simulink library "libturbines"  (R2025b)
settings: Solver=ode45  StartTime=0.0  StopTime=10.0  RelTol=1e-3  EnableMultiTasking=on
undefined symbols (not defined in the file): DiscIntNeverNeededParam, dt, faultOptions, noiseFlag
libraries: simulink x57, $bdroot x3
(part 2 of 5)

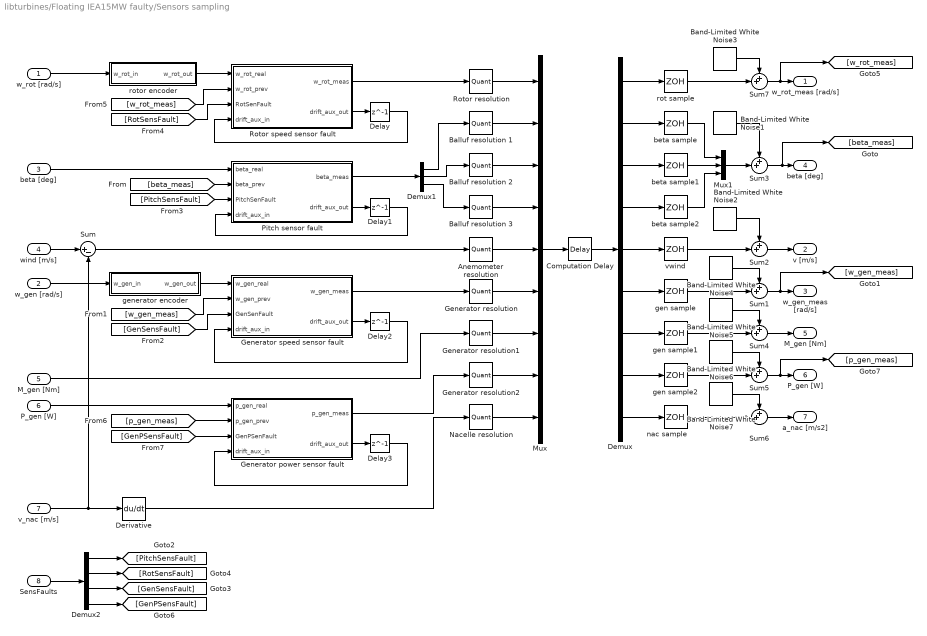
== system libturbines/Floating IEA15MW faulty/Sensors sampling ==
  "w_rot [rad/s] " : Inport
  w_gen [rad/s] : Inport  Port=2
  "beta [deg] " : Inport  Port=3
  wind [m/s] : Inport  Port=4
  "M_gen [Nm] " : Inport  Port=5
  "P_gen [W] " : Inport  Port=6
  "v_nac [m/s] " : Inport  Port=7
  SensFaults : Inport  Port=8
  Anemometer resolution : Quantizer  QuantizationInterval=wt.meas.aneres
  Balluf resolution 1 : Quantizer  QuantizationInterval=wt.meas.pitchres
  Balluf resolution 2 : Quantizer  QuantizationInterval=wt.meas.pitchres
  Balluf resolution 3 : Quantizer  QuantizationInterval=wt.meas.pitchres
  Band-Limited White Noise1 : simulink/Sources/Band-Limited White Noise  Cov=noiseFlag*wt.meas.pitchnoise  Ts=dt  seed=floor(10000*rand(1,3))
  Band-Limited White Noise2 : simulink/Sources/Band-Limited White Noise  Cov=noiseFlag*wt.meas.anenoise  Ts=dt  seed=floor(10000*rand(1))
  Band-Limited White Noise3 : simulink/Sources/Band-Limited White Noise  Cov=noiseFlag*wt.meas.rotSpdnoise  Ts=dt  seed=floor(10000*rand(1))
  Band-Limited White Noise4 : simulink/Sources/Band-Limited White Noise  Cov=noiseFlag*wt.meas.genSpdnoise  Ts=dt  seed=floor(10000*rand(1))
  Band-Limited White Noise5 : simulink/Sources/Band-Limited White Noise  Cov=noiseFlag*wt.meas.genTrqnoise  Ts=dt  seed=floor(10000*rand(1))
  Band-Limited White Noise6 : simulink/Sources/Band-Limited White Noise  Cov=noiseFlag*wt.meas.genPwrnoise  Ts=dt  seed=floor(10000*rand(1))
  Band-Limited White Noise7 : simulink/Sources/Band-Limited White Noise  Cov=noiseFlag*wt.meas.nacAccnoise  Ts=dt  seed=floor(10000*rand(1))
  Computation Delay : TransportDelay  DelayTime=wt.meas.delay  InitialOutput=[wt.rotor.ini wt.pitch.ini wt.pitch.ini wt.pitch.ini 0 wt.gen.ini 0 0 0]
  Delay{,1..3} (4 alike) : Delay  DelayLength=1  InitialCondition=0
  Demux : Demux  Outputs=9
  Demux1 : Demux  Outputs=3
  Demux2 : Demux
  Derivative : Derivative
  Generator power sensor fault : MATLAB Function  TreatAsAtomicUnit=on
  Generator resolution : Quantizer  QuantizationInterval=wt.meas.genres
  Generator resolution1 : Quantizer  QuantizationInterval=wt.meas.genres
  Generator resolution2 : Quantizer  QuantizationInterval=wt.meas.genres
  Generator speed sensor fault : MATLAB Function  TreatAsAtomicUnit=on
  Mux : Mux  Inputs=9
  Mux1 : Mux  Inputs=3
  Nacelle resolution : Quantizer  QuantizationInterval=wt.meas.nacres
  Pitch sensor fault : MATLAB Function  TreatAsAtomicUnit=on
  Rotor resolution : Quantizer  QuantizationInterval=wt.meas.rotres
  Rotor speed sensor fault : MATLAB Function  TreatAsAtomicUnit=on
  Sum : Sum  Inputs=|+-
  Sum{1..7} (7 alike) : Sum  Inputs=++|
  beta sample : ZeroOrderHold  SampleTime=wt.meas.Ts
  beta sample1 : ZeroOrderHold  SampleTime=wt.meas.Ts
  beta sample2 : ZeroOrderHold  SampleTime=wt.meas.Ts
  gen sample : ZeroOrderHold  SampleTime=wt.meas.Ts
  gen sample1 : ZeroOrderHold  SampleTime=wt.meas.Ts
  gen sample2 : ZeroOrderHold  SampleTime=wt.meas.Ts
  generator encoder : Subsystem
  nac sample : ZeroOrderHold  SampleTime=wt.meas.Ts
  rot sample : ZeroOrderHold  SampleTime=wt.meas.Ts
  rotor encoder : Subsystem
  vwind : ZeroOrderHold  SampleTime=wt.meas.Ts
  w_rot_meas [rad/s] : Outport  InitialOutput=0
  v [m/s] : Outport  Port=2  InitialOutput=0
  w_gen_meas [rad/s] : Outport  Port=3  InitialOutput=0
  beta [deg] : Outport  Port=4  InitialOutput=0
  M_gen [Nm] : Outport  Port=5  InitialOutput=0
  P_gen [W] : Outport  Port=6  InitialOutput=0
  a_nac [m/s2] : Outport  Port=7  InitialOutput=0
  wires:
  [p_gen_meas] -> Generator power sensor fault/2(p_gen_prev)
  Generator power sensor fault/1(p_gen_meas) -> Generator resolution2/1
  "P_gen [W] "/1 -> Generator power sensor fault/1(p_gen_real)
  Generator power sensor fault/2(drift_aux_out) -> Delay3/1
  [GenPSensFault] -> Generator power sensor fault/3(GenPSenFault)
  Delay3/1 -> Generator power sensor fault/4(drift_aux_in)
  Demux2/4 -> [GenPSensFault]
  wind [m/s]/1 -> Sum/1
  Sum/1 -> Anemometer resolution/1
  Band-Limited White Noise3/1 -> Sum7/1
  Band-Limited White Noise1/1 -> Sum3/1
  Band-Limited White Noise2/1 -> Sum2/1
  Band-Limited White Noise4/1 -> Sum1/1
  Sum7/1 -> w_rot_meas [rad/s]/1, [w_rot_meas]
  rot sample/1 -> Sum7/2
  Sum3/1 -> beta [deg]/1, [beta_meas]
  Mux1/1 -> Sum3/2
  vwind/1 -> Sum2/2
  Sum2/1 -> v [m/s]/1
  gen sample/1 -> Sum1/2
  Sum1/1 -> w_gen_meas [rad/s]/1, [w_gen_meas]
  Demux/9 -> nac sample/1
  Demux/8 -> gen sample2/1
  Demux/7 -> gen sample1/1
  gen sample2/1 -> Sum5/2
  Sum5/1 -> P_gen [W]/1, [p_gen_meas]
  gen sample1/1 -> Sum4/2
  nac sample/1 -> Sum6/2
  Band-Limited White Noise6/1 -> Sum5/1
  Band-Limited White Noise7/1 -> Sum6/1
  Sum6/1 -> a_nac [m/s2]/1
  Sum4/1 -> M_gen [Nm]/1
  Band-Limited White Noise5/1 -> Sum4/1
  Generator resolution2/1 -> Mux/8
  Nacelle resolution/1 -> Mux/9
  Generator resolution1/1 -> Mux/7
  Derivative/1 -> Nacelle resolution/1
  "v_nac [m/s] "/1 -> Sum/2, Derivative/1
  "M_gen [Nm] "/1 -> Generator resolution1/1
  Delay2/1 -> Generator speed sensor fault/4(drift_aux_in)
  Generator speed sensor fault/2(drift_aux_out) -> Delay2/1
  Delay1/1 -> Pitch sensor fault/4(drift_aux_in)
  Pitch sensor fault/2(drift_aux_out) -> Delay1/1
  Delay/1 -> Rotor speed sensor fault/4(drift_aux_in)
  Rotor speed sensor fault/2(drift_aux_out) -> Delay/1
  Demux2/3 -> [GenSensFault]
  Demux2/2 -> [RotSensFault]
  [w_rot_meas] -> Rotor speed sensor fault/2(w_rot_prev)
  [RotSensFault] -> Rotor speed sensor fault/3(RotSenFault)
  [PitchSensFault] -> Pitch sensor fault/3(PitchSenFault)
  [GenSensFault] -> Generator speed sensor fault/3(GenSenFault)
  Demux2/1 -> [PitchSensFault]
  SensFaults/1 -> Demux2/1
  rotor encoder/1(w_rot_out) -> Rotor speed sensor fault/1(w_rot_real)
  Rotor speed sensor fault/1(w_rot_meas) -> Rotor resolution/1
  "w_rot [rad/s] "/1 -> rotor encoder/1(w_rot_in)
  generator encoder/1(w_gen_out) -> Generator speed sensor fault/1(w_gen_real)
  w_gen [rad/s]/1 -> generator encoder/1(w_gen_in)
  [beta_meas] -> Pitch sensor fault/2(beta_prev)
  [w_gen_meas] -> Generator speed sensor fault/2(w_gen_prev)
  Generator speed sensor fault/1(w_gen_meas) -> Generator resolution/1
  Balluf resolution 3/1 -> Mux/4
  Balluf resolution 2/1 -> Mux/3
  Demux/3 -> beta sample1/1
  Demux/4 -> beta sample2/1
  "beta [deg] "/1 -> Pitch sensor fault/1(beta_real)
  Pitch sensor fault/1(beta_meas) -> Demux1/1
  Balluf resolution 1/1 -> Mux/2
  Demux/2 -> beta sample/1
  beta sample2/1 -> Mux1/3
  Demux/1 -> rot sample/1
  beta sample/1 -> Mux1/1
  Demux1/3 -> Balluf resolution 3/1
  Computation Delay/1 -> Demux/1
  Mux/1 -> Computation Delay/1
  Demux/5 -> vwind/1
  Anemometer resolution/1 -> Mux/5
  Demux/6 -> gen sample/1
  Demux1/2 -> Balluf resolution 2/1
  Generator resolution/1 -> Mux/6
  Rotor resolution/1 -> Mux/1
  Demux1/1 -> Balluf resolution 1/1
  beta sample1/1 -> Mux1/2

== system libturbines/Floating IEA15MW faulty/Tower deflection  ==
  F_t [N] : Inport
  F_t*h : Gain  Gain=wt.tower.height  SaturateOnIntegerOverflow=on  OutDataTypeStr=Inherit: Same as input  ParamDataTypeStr=Inherit: Same as input
  Tower1 : Subsystem  mask(Tower (thrustwise)){mtop=wt.top.mass, mtow=wt.tower.mass, ftowY=wt.tower.eigfreq, dampY=wt.tower.damp}
      mask prompts: mtop "Mass of towertop [kg]"; mtow "Aequivalent tower mass [kg]"; ftowY "Tower eigenfrequency [Hz]"; dampY "Damping coefficient"
      mask help: Thrustwise dynamics of the tower
      mask init: same as libturbines/Floating IEA15MW/Tower /Tower1
      mask Help: The thrustwise tower dynamics are modelled as a linear oscillator
  v_nac [m/s] : Outport
  M_tow [Nm] : Outport  Port=2
  wires:
  Tower1/1(vnac [m/s]) -> v_nac [m/s]/1
  F_t [N]/1 -> Tower1/1(FT [Nm])
  F_t*h/1 -> M_tow [Nm]/1
  Tower1/2(F_tow [N]) -> F_t*h/1

== system libturbines/Floating IEA3.4MW/Aerodynamics ==
  note: tip speed
      | [m/s]
  w_rot [rad/s] : Inport
  beta [deg] : Inport  Port=2
  v_rot [m/s] : Inport  Port=3
  C_P & C_T tables1 : $bdroot/Floating NREL5MW faulty/Aerodynamics/Blade 1/C_P & C_T tables  SystemSampleTime=-1  VariantActivationTime=update diagram  EmptyChoice=off  PassThrough=off  PassThroughVariantControl=(default)  EmptyChoiceVariantControl=(default)  AllowFlexibleInterface=on  Latency=0  AutoFrameSizeCalculation=off
  Math Function : Math  Operator=square  SignedPower=on
  Product : Product  InputSameDT=on  SaturateOnIntegerOverflow=on  OutDataTypeStr=Inherit: Same as first input
  Product1 : Product  Inputs=**/  InputSameDT=on  SaturateOnIntegerOverflow=on  OutDataTypeStr=Inherit: Same as first input
  Product2 : Product  InputSameDT=on  SaturateOnIntegerOverflow=on  OutDataTypeStr=Inherit: Same as first input
  Product3 : Product  Inputs=/*  InputSameDT=on  SaturateOnIntegerOverflow=on  OutDataTypeStr=Inherit: Same as first input
  rho/2*A : Gain  Gain=env.rho*.5* pi * wt.rotor.radius^2  SaturateOnIntegerOverflow=on  OutDataTypeStr=Inherit: Same as input  ParamDataTypeStr=Inherit: Same as input
  rotor radius : Gain  Gain=wt.rotor.radius  SaturateOnIntegerOverflow=on  OutDataTypeStr=Inherit: Same as input  ParamDataTypeStr=Inherit: Same as input
  M_rot [Nm] : Outport
  F_t [N] : Outport  Port=2
  C_T : Outport  Port=3
  wires:
  rho/2*A/1 -> Product/1, Product2/2
  C_P & C_T tables1/1 -> Product/2, C_T/1
  Product3/1 -> C_P & C_T tables1/2
  w_rot [rad/s]/1 -> Product1/3, rotor radius/1
  v_rot [m/s]/1 -> Product2/1, Product3/1, Math Function/1
  Math Function/1 -> rho/2*A/1
  rotor radius/1 -> Product3/2
  C_P & C_T tables1/2 -> Product1/1
  beta [deg]/1 -> C_P & C_T tables1/1
  Product/1 -> F_t [N]/1
  Product1/1 -> M_rot [Nm]/1
  Product2/1 -> Product1/2

== system libturbines/Floating IEA3.4MW/Controller ==
  P_dem [W] : Inport
  w_gen_meas [m/s] : Inport  Port=2
  beta_meas [deg] : Inport  Port=3
  Generator efficiency compensation : Gain  Gain=1/wt.ctrl.gen.effeciency
  Limit power to rated : Saturate  UpperLimit=wt.ctrl.p_rated  LowerLimit=0
  Measurement filter (low pass) : DiscreteStateSpace  A=wt.ctrl.alpha  B=1-wt.ctrl.alpha  C=wt.ctrl.alpha  D=1-wt.ctrl.alpha  InitialCondition=wt.ctrl.gen.ini  SampleTime=wt.ctrl.Ts
  Pitch controller : Subsystem  TreatAsAtomicUnit=on
  Rate Limiter : RateLimiter  RisingSlewLimit=wt.ctrl.torq.ratelim  FallingSlewLimit=-wt.ctrl.torq.ratelim  SampleTimeMode=inherited  InitialCondition=wt.ctrl.torq.ini
  Rated speed : Constant  Value=wt.ctrl.gen.rated
  Region check : Subsystem
  Sample output : ZeroOrderHold  SampleTime=wt.ctrl.Ts
  Sample power demand : ZeroOrderHold  SampleTime=wt.ctrl.Ts
  Saturation : Saturate  UpperLimit=wt.ctrl.torq.lim  LowerLimit=0
  Sum : Sum  Inputs=+-|
  Torque - speed lookup table : Lookup  InputValues=wt.ctrl.torq.wg  Table=wt.ctrl.torq.M  LookUpMeth=Interpolation-Use End Values  SaturateOnIntegerOverflow=off
  Zero-Order Hold : ZeroOrderHold  SampleTime=wt.ctrl.Ts
  beta_ref [deg] : Outport
  M_g_ref [W] : Outport  Port=2
  wires:
  Region check/2(Enable pitch controller) -> Pitch controller/Enable
  Sum/1 -> Pitch controller/1(w_gen_diff)
  Rated speed/1 -> Sum/1
  Sample power demand/1 -> Generator efficiency compensation/1
  Rate Limiter/1 -> Sample output/1
  Generator efficiency compensation/1 -> Limit power to rated/1
  Sample output/1 -> M_g_ref [W]/1
  Zero-Order Hold/1 -> beta_ref [deg]/1
  Limit power to rated/1 -> Region check/3(p_dem), Pitch controller/2(P_dem)
  Region check/1(Torque_ref) -> Saturation/1
  P_dem [W]/1 -> Sample power demand/1
  Torque - speed lookup table/1 -> Region check/1(Torque_dem)  "Desired Torque"
  Saturation/1 -> Rate Limiter/1
  Measurement filter (low pass)/1 -> Sum/2, Region check/2(w_gen), Torque - speed lookup table/1  "Filtered generator speed"
  w_gen_meas [m/s]/1 -> Measurement filter (low pass)/1
  Pitch controller/1(beta_ref [deg]) -> Zero-Order Hold/1, Region check/4(pitch command)
  beta_meas [deg]/1 -> Pitch controller/3(beta_meas [deg])

== system libturbines/Floating IEA3.4MW/Drive Train ==
  M_rot [Nm] : Inport
  M_gen [Nm] : Inport  Port=2
  Demux : Demux  Outputs=3
  Drive train dynamics : StateSpace  A=wt.dt.ssA  B=wt.dt.ssB  C=wt.dt.ssC  D=wt.dt.ssD  InitialCondition=[wt.rotor.ini;wt.gen.ini;0]
  Mux : Mux  Inputs=2
  w_rot [rad/s] : Outport
  w_gen [rad/s] : Outport  Port=2
  M_shaft [Nm] : Outport  Port=3
  wires:
  Mux/1 -> Drive train dynamics/1
  M_rot [Nm]/1 -> Mux/1
  M_gen [Nm]/1 -> Mux/2
  Drive train dynamics/1 -> Demux/1
  Demux/1 -> w_rot [rad/s]/1
  Demux/2 -> w_gen [rad/s]/1
  Demux/3 -> M_shaft [Nm]/1

== system libturbines/Floating IEA3.4MW/Generator simple ==
  w_gen [rad/s] : Inport
  M_g_ref [W] : Inport  Port=2
  Constant : Constant  Value=wt.gen.timeconstant
  Divide1 : Product  Inputs=*/
  Generator efficiency : Gain  Gain=wt.gen.effeciency
  Multiply : Product  Inputs=**
  Sum : Sum  Inputs=|+-
  Torque Integrator : Integrator  InitialCondition=wt.gen.torq.ini
  M_gen [Nm] : Outport
  P_out [W] : Outport  Port=2
  wires:
  Constant/1 -> Divide1/2
  Divide1/1 -> Torque Integrator/1
  Generator efficiency/1 -> P_out [W]/1
  Multiply/1 -> Generator efficiency/1
  M_g_ref [W]/1 -> Sum/1
  w_gen [rad/s]/1 -> Multiply/2
  Torque Integrator/1 -> M_gen [Nm]/1, Sum/2, Multiply/1
  Sum/1 -> Divide1/1

== system libturbines/Floating IEA3.4MW/Hydrodynamics ==
  F_t [N] : Inport
  F_ex : Inport  Port=2
  Gain : Gain  Gain=plat.nF2pT  Multiplication=Matrix(K*u)
  Gain2 : Gain  Gain=plat.pM2nM_surge  Multiplication=Matrix(K*u)
  Gain3 : Gain  Gain=plat.pM2nM_pitch  Multiplication=Matrix(K*u)
  Platform hydrodynamics SS system : StateSpace  A=plat.HydSys.a  B=plat.HydSys.b  C=plat.HydSys.c  D=plat.HydSys.d  InitialCondition=0
  Sum : Sum  Inputs=++|
  Sum2 : Sum  Inputs=+|+
  v_nac_hyd [m/s] : Outport
  wires:
  F_ex/1 -> Sum/2
  Sum/1 -> Platform hydrodynamics SS system/1
  Sum2/1 -> v_nac_hyd [m/s]/1
  Platform hydrodynamics SS system/1 -> Gain3/1, Gain2/1
  Gain2/1 -> Sum2/1
  Gain3/1 -> Sum2/2
  Gain/1 -> Sum/1
  F_t [N]/1 -> Gain/1

== system libturbines/Floating IEA3.4MW/Pitch Actuator ==
  beta_ref [deg] : Inport
  Pitch system : StateSpace  A=wt.pitch.ssA  B=wt.pitch.ssB  C=wt.pitch.ssC  D=wt.pitch.ssD  InitialCondition=0
  beta [deg] : Outport
  wires:
  beta_ref [deg]/1 -> Pitch system/1
  Pitch system/1 -> beta [deg]/1

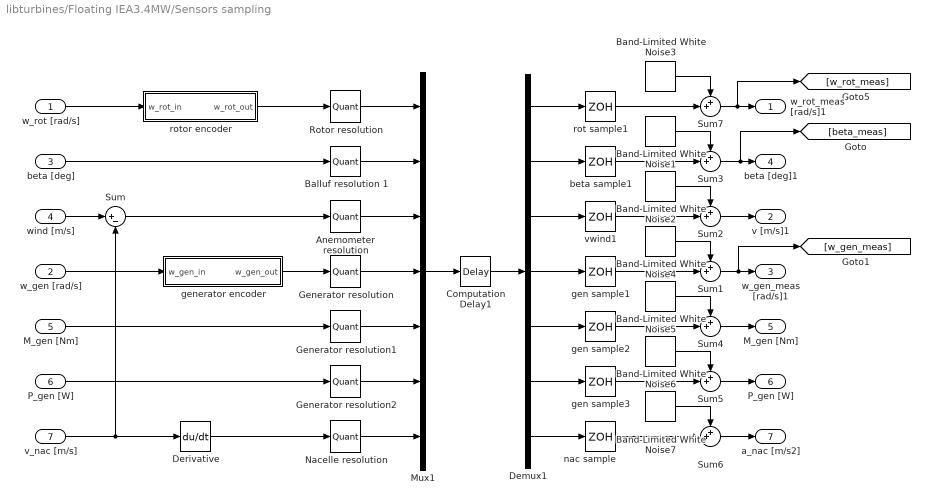
== system libturbines/Floating IEA3.4MW/Sensors sampling ==
  "w_rot [rad/s] " : Inport
  w_gen [rad/s] : Inport  Port=2
  "beta [deg] " : Inport  Port=3
  wind [m/s] : Inport  Port=4
  "M_gen [Nm] " : Inport  Port=5
  "P_gen [W] " : Inport  Port=6
  "v_nac [m/s] " : Inport  Port=7
  Anemometer resolution : Quantizer  QuantizationInterval=wt.meas.aneres
  Balluf resolution 1 : Quantizer  QuantizationInterval=wt.meas.pitchres
  Band-Limited White Noise1 : simulink/Sources/Band-Limited White Noise  Cov=noiseFlag*wt.meas.pitchnoise  Ts=dt  seed=floor(10000*rand(1))
  Band-Limited White Noise2 : simulink/Sources/Band-Limited White Noise  Cov=noiseFlag*wt.meas.anenoise  Ts=dt  seed=floor(10000*rand(1))
  Band-Limited White Noise3 : simulink/Sources/Band-Limited White Noise  Cov=noiseFlag*wt.meas.rotSpdnoise  Ts=dt  seed=floor(10000*rand(1))
  Band-Limited White Noise4 : simulink/Sources/Band-Limited White Noise  Cov=noiseFlag*wt.meas.genSpdnoise  Ts=dt  seed=floor(10000*rand(1))
  Band-Limited White Noise5 : simulink/Sources/Band-Limited White Noise  Cov=noiseFlag*wt.meas.genTrqnoise  Ts=dt  seed=floor(10000*rand(1))
  Band-Limited White Noise6 : simulink/Sources/Band-Limited White Noise  Cov=noiseFlag*wt.meas.genPwrnoise  Ts=dt  seed=floor(10000*rand(1))
  Band-Limited White Noise7 : simulink/Sources/Band-Limited White Noise  Cov=noiseFlag*wt.meas.nacAccnoise  Ts=dt  seed=floor(10000*rand(1))
  Computation Delay1 : TransportDelay  DelayTime=wt.meas.delay  InitialOutput=[wt.rotor.ini wt.pitch.ini 0 wt.gen.ini 0 0 0]
  Demux1 : Demux  Outputs=7
  Derivative : Derivative
  Generator resolution : Quantizer  QuantizationInterval=wt.meas.genres
  Generator resolution1 : Quantizer  QuantizationInterval=wt.meas.genres
  Generator resolution2 : Quantizer  QuantizationInterval=wt.meas.genres
  Mux1 : Mux  Inputs=7
  Nacelle resolution : Quantizer  QuantizationInterval=wt.meas.nacres
  Rotor resolution : Quantizer  QuantizationInterval=wt.meas.rotres
  Sum : Sum  Inputs=|+-
  Sum{1..7} (7 alike) : Sum  Inputs=++|
  beta sample1 : ZeroOrderHold  SampleTime=wt.meas.Ts
  gen sample1 : ZeroOrderHold  SampleTime=wt.meas.Ts
  gen sample2 : ZeroOrderHold  SampleTime=wt.meas.Ts
  gen sample3 : ZeroOrderHold  SampleTime=wt.meas.Ts
  generator encoder : Subsystem
  nac sample : ZeroOrderHold  SampleTime=wt.meas.Ts
  rot sample1 : ZeroOrderHold  SampleTime=wt.meas.Ts
  rotor encoder : Subsystem
  vwind1 : ZeroOrderHold  SampleTime=wt.meas.Ts
  w_rot_meas [rad/s]1 : Outport  InitialOutput=0
  v [m/s]1 : Outport  Port=2  InitialOutput=0
  w_gen_meas [rad/s]1 : Outport  Port=3  InitialOutput=0
  beta [deg]1 : Outport  Port=4  InitialOutput=0
  M_gen [Nm] : Outport  Port=5  InitialOutput=0
  P_gen [W] : Outport  Port=6  InitialOutput=0
  a_nac [m/s2] : Outport  Port=7  InitialOutput=0
  wires:
  Sum/1 -> Anemometer resolution/1
  wind [m/s]/1 -> Sum/1
  "M_gen [Nm] "/1 -> Generator resolution1/1
  "P_gen [W] "/1 -> Generator resolution2/1
  Derivative/1 -> Nacelle resolution/1
  Nacelle resolution/1 -> Mux1/7
  Generator resolution2/1 -> Mux1/6
  Generator resolution1/1 -> Mux1/5
  Demux1/3 -> vwind1/1
  Demux1/4 -> gen sample1/1
  Demux1/5 -> gen sample2/1
  Demux1/6 -> gen sample3/1
  Demux1/7 -> nac sample/1
  "v_nac [m/s] "/1 -> Derivative/1, Sum/2
  Generator resolution/1 -> Mux1/4
  Anemometer resolution/1 -> Mux1/3
  Balluf resolution 1/1 -> Mux1/2
  Band-Limited White Noise2/1 -> Sum2/1
  gen sample2/1 -> Sum4/2
  Sum1/1 -> w_gen_meas [rad/s]1/1, [w_gen_meas]
  Sum5/1 -> P_gen [W]/1
  gen sample3/1 -> Sum5/2
  Band-Limited White Noise1/1 -> Sum3/1
  nac sample/1 -> Sum6/2
  Sum4/1 -> M_gen [Nm]/1
  Sum6/1 -> a_nac [m/s2]/1
  vwind1/1 -> Sum2/2
  Sum7/1 -> w_rot_meas [rad/s]1/1, [w_rot_meas]
  Band-Limited White Noise4/1 -> Sum1/1
  Band-Limited White Noise5/1 -> Sum4/1
  gen sample1/1 -> Sum1/2
  Band-Limited White Noise3/1 -> Sum7/1
  rot sample1/1 -> Sum7/2
  Mux1/1 -> Computation Delay1/1
  Sum3/1 -> beta [deg]1/1, [beta_meas]
  Sum2/1 -> v [m/s]1/1
  Band-Limited White Noise6/1 -> Sum5/1
  Band-Limited White Noise7/1 -> Sum6/1
  Demux1/2 -> beta sample1/1
  Demux1/1 -> rot sample1/1
  beta sample1/1 -> Sum3/2
  Computation Delay1/1 -> Demux1/1
  "beta [deg] "/1 -> Balluf resolution 1/1
  Rotor resolution/1 -> Mux1/1
  generator encoder/1(w_gen_out) -> Generator resolution/1
  w_gen [rad/s]/1 -> generator encoder/1(w_gen_in)
  "w_rot [rad/s] "/1 -> rotor encoder/1(w_rot_in)
  rotor encoder/1(w_rot_out) -> Rotor resolution/1

== system libturbines/Floating IEA3.4MW/Tower  ==
  F_t [N] : Inport
  F_t*h : Gain  Gain=wt.tower.height  SaturateOnIntegerOverflow=on  OutDataTypeStr=Inherit: Same as input  ParamDataTypeStr=Inherit: Same as input
  Tower1 : Subsystem  mask(Tower (thrustwise)){mtop=wt.top.mass, mtow=wt.tower.mass, ftowY=wt.tower.eigfreq, dampY=wt.tower.damp}
      mask prompts: mtop "Mass of towertop [kg]"; mtow "Aequivalent tower mass [kg]"; ftowY "Tower eigenfrequency [Hz]"; dampY "Damping coefficient"
      mask help: Thrustwise dynamics of the tower
      mask init: same as libturbines/Floating IEA15MW/Tower /Tower1
      mask Help: The thrustwise tower dynamics are modelled as a linear oscillator
  M_tow [Nm] : Outport
  v_nac [m/s] : Outport  Port=2
  wires:
  Tower1/2(F_tow [N]) -> F_t*h/1
  F_t*h/1 -> M_tow [Nm]/1
  F_t [N]/1 -> Tower1/1(FT [Nm])
  Tower1/1(vnac [m/s]) -> v_nac [m/s]/1

== system libturbines/Floating IEA3.4MW faulty/Aerodynamics ==
  w_rot [rad/s] : Inport
  beta [deg] : Inport  Port=2
  v_rot [m/s] : Inport  Port=3
  Blade 1 : Subsystem
  Blade 2 : Subsystem  AncestorBlock=libturbines/Floating faulty NREL5MW1/Aerodynamics/Blade 1
  Blade 3 : Subsystem  AncestorBlock=libturbines/Floating faulty NREL5MW1/Aerodynamics/Blade 1
  Demux : Demux  Outputs=3
  Sum : Sum  Inputs=+++
  Sum1 : Sum  Inputs=+++
  Sum2 : Sum  Inputs=+++
  M_rot [Nm] : Outport
  F_t [N] : Outport  Port=2
  C_T : Outport  Port=3
  wires:
  Demux/2 -> Blade 2/2(beta [deg])
  Demux/3 -> Blade 3/2(beta [deg])
  Demux/1 -> Blade 1/2(beta [deg])
  beta [deg]/1 -> Demux/1
  Blade 2/2(C_T) -> Sum1/2
  Blade 2/1(F_t [N]) -> Sum/2
  Blade 1/2(C_T) -> Sum1/1
  Blade 1/1(F_t [N]) -> Sum/1
  Blade 1/3(M_rot [Nm]) -> Sum2/1
  Blade 3/2(C_T) -> Sum1/3
  Blade 3/1(F_t [N]) -> Sum/3
  Blade 3/3(M_rot [Nm]) -> Sum2/3
  Blade 2/3(M_rot [Nm]) -> Sum2/2
  Sum1/1 -> C_T/1
  Sum2/1 -> M_rot [Nm]/1
  Sum/1 -> F_t [N]/1
  w_rot [rad/s]/1 -> Blade 1/3(w_rot [rad/s]), Blade 2/3(w_rot [rad/s]), Blade 3/3(w_rot [rad/s])
  v_rot [m/s]/1 -> Blade 1/1(v_rot [m/s]), Blade 2/1(v_rot [m/s]), Blade 3/1(v_rot [m/s])

== system libturbines/Floating IEA3.4MW faulty/Controller ==
  P_dem [W] : Inport
  w_gen_meas [m/s] : Inport  Port=2
  beta_meas [deg] : Inport  Port=3
  Gain : Gain  Gain=[1 0 0]  Multiplication=Matrix(K*u) (u vector)
  Generator efficiency compensation : Gain  Gain=1/wt.ctrl.gen.effeciency
  Limit power to rated : Saturate  UpperLimit=wt.ctrl.p_rated  LowerLimit=0
  Measurement filter (low pass) : DiscreteStateSpace  A=wt.ctrl.alpha  B=1-wt.ctrl.alpha  C=wt.ctrl.alpha  D=1-wt.ctrl.alpha  InitialCondition=wt.ctrl.gen.ini  SampleTime=wt.ctrl.Ts
  Pitch controller : Subsystem  TreatAsAtomicUnit=on
  Rate Limiter : RateLimiter  RisingSlewLimit=wt.ctrl.torq.ratelim  FallingSlewLimit=-wt.ctrl.torq.ratelim  SampleTimeMode=inherited  InitialCondition=wt.ctrl.torq.ini
  Rated speed : Constant  Value=wt.ctrl.gen.rated
  Region check : Subsystem
  Sample output : ZeroOrderHold  SampleTime=wt.ctrl.Ts
  Sample power demand : ZeroOrderHold  SampleTime=wt.ctrl.Ts
  Saturation : Saturate  UpperLimit=wt.ctrl.torq.lim  LowerLimit=0
  Sum : Sum  Inputs=+-|
  Torque - speed lookup table : Lookup  InputValues=wt.ctrl.torq.wg  Table=wt.ctrl.torq.M  LookUpMeth=Interpolation-Use End Values  SaturateOnIntegerOverflow=off
  Zero-Order Hold : ZeroOrderHold  SampleTime=wt.ctrl.Ts
  beta_ref [deg] : Outport
  T_g_ref [W] : Outport  Port=2
  wires:
  beta_meas [deg]/1 -> Pitch controller/3(beta_meas [deg])
  Gain/1 -> Region check/4(pitch command)
  w_gen_meas [m/s]/1 -> Measurement filter (low pass)/1
  Measurement filter (low pass)/1 -> Torque - speed lookup table/1, Region check/2(w_gen), Sum/2  "Filtered generator speed"
  Saturation/1 -> Rate Limiter/1
  Pitch controller/1(beta_ref [deg]) -> Zero-Order Hold/1, Gain/1
  Torque - speed lookup table/1 -> Region check/1(Torque_dem)  "Desired Torque"
  P_dem [W]/1 -> Sample power demand/1
  Region check/1(Torque_ref) -> Saturation/1
  Limit power to rated/1 -> Pitch controller/2(P_dem), Region check/3(p_dem)
  Zero-Order Hold/1 -> beta_ref [deg]/1
  Sample output/1 -> T_g_ref [W]/1
  Generator efficiency compensation/1 -> Limit power to rated/1
  Rate Limiter/1 -> Sample output/1
  Sample power demand/1 -> Generator efficiency compensation/1
  Rated speed/1 -> Sum/1
  Sum/1 -> Pitch controller/1(w_gen_diff)
  Region check/2(Enable pitch controller) -> Pitch controller/Enable

== system libturbines/Floating IEA3.4MW faulty/Drive Train ==
  M_rot [Nm] : Inport
  M_gen [Nm] : Inport  Port=2
  Demux : Demux  Outputs=3
  Drive train dynamics : StateSpace  A=wt.dt.ssA  B=wt.dt.ssB  C=wt.dt.ssC  D=wt.dt.ssD  InitialCondition=[wt.rotor.ini;wt.gen.ini;0]
  Mux : Mux  Inputs=2
  w_rot [rad/s] : Outport
  w_gen [rad/s] : Outport  Port=2
  M_shaft [Nm] : Outport  Port=3
  wires:
  Demux/3 -> M_shaft [Nm]/1
  Demux/2 -> w_gen [rad/s]/1
  Demux/1 -> w_rot [rad/s]/1
  Drive train dynamics/1 -> Demux/1
  M_gen [Nm]/1 -> Mux/2
  M_rot [Nm]/1 -> Mux/1
  Mux/1 -> Drive train dynamics/1

== system libturbines/Floating IEA3.4MW faulty/Generator simple ==
  w_gen [rad/s] : Inport
  T_g_ref [W] : Inport  Port=2
  GenActFault : Inport  Port=3
  Constant : Constant  Value=wt.gen.timeconstant
  Delay : Delay  DelayLength=1  InitialCondition=0
  Delay1 : Delay  DelayLength=1  InitialCondition=0
  Demux : Demux  Outputs=2
  Divide1 : Product  Inputs=*/
  Generator efficiency : Gain  Gain=wt.gen.effeciency
  Generator fault : MATLAB Function  TreatAsAtomicUnit=on
  Generator fault type 3 : MATLAB Function  TreatAsAtomicUnit=on
  Multiply : Product  Inputs=**
  Product : Product
  Sum : Sum  Inputs=|+-
  Torque Integrator : Integrator  InitialCondition=wt.gen.torq.ini
  M_gen [Nm] : Outport
  P_out [W] : Outport  Port=2
  wires:
  Delay1/1 -> Generator fault/4(drift_aux_in)
  Generator fault/2(drift_aux_out) -> Delay1/1
  Delay/1 -> Generator fault/3(torque_prev)
  Sum/1 -> Divide1/1
  Product/1 -> Divide1/2
  Demux/2 -> Product/1
  Constant/1 -> Product/2
  Generator fault/1(torque_real) -> M_gen [Nm]/1, Delay/1, Multiply/1
  Demux/1 -> Generator fault/1(GenActFault)
  Generator fault type 3/1(out) -> Demux/1
  GenActFault/1 -> Generator fault type 3/1(GenActFault)
  w_gen [rad/s]/1 -> Multiply/2
  Torque Integrator/1 -> Sum/2, Generator fault/2(torque)
  T_g_ref [W]/1 -> Sum/1
  Multiply/1 -> Generator efficiency/1
  Generator efficiency/1 -> P_out [W]/1
  Divide1/1 -> Torque Integrator/1

== system libturbines/Floating IEA3.4MW faulty/Hydrodynamics ==
  F_t [N] : Inport
  F_ex : Inport  Port=2
  Gain : Gain  Gain=plat.nF2pT  Multiplication=Matrix(K*u)
  Gain2 : Gain  Gain=plat.pM2nM_surge  Multiplication=Matrix(K*u)
  Gain3 : Gain  Gain=plat.pM2nM_pitch  Multiplication=Matrix(K*u)
  Platform hydrodynamics SS system : StateSpace  A=plat.HydSys.a  B=plat.HydSys.b  C=plat.HydSys.c  D=plat.HydSys.d  InitialCondition=0
  Sum : Sum  Inputs=++|
  Sum2 : Sum  Inputs=+|+
  v_nac_hyd [m/s] : Outport
  wires:
  F_t [N]/1 -> Gain/1
  Gain/1 -> Sum/1
  Gain3/1 -> Sum2/2
  Gain2/1 -> Sum2/1
  Platform hydrodynamics SS system/1 -> Gain2/1, Gain3/1
  Sum2/1 -> v_nac_hyd [m/s]/1
  Sum/1 -> Platform hydrodynamics SS system/1
  F_ex/1 -> Sum/2

== system libturbines/Floating IEA3.4MW faulty/Pitch Actuator ==
  beta_ref [deg] : Inport
  PitchActFault : Inport  Port=2
  Delay1 : Delay  DelayLength=1  InitialCondition=0
  Delay2 : Delay  DelayLength=1  InitialCondition=0
  Pitch actuator fault : MATLAB Function  TreatAsAtomicUnit=on
  Pitch subsystems : Subsystem
  beta [deg] : Outport
  wires:
  Delay1/1 -> Pitch actuator fault/2(beta_prev)
  Delay2/1 -> Pitch actuator fault/4(drift_aux_in)
  Pitch actuator fault/2(drift_aux_out) -> Delay2/1
  Pitch subsystems/1(beta [deg]) -> Pitch actuator fault/1(beta)
  Pitch actuator fault/1(beta_real) -> beta [deg]/1, Delay1/1
  beta_ref [deg]/1 -> Pitch subsystems/1(beta_ref [deg])
  PitchActFault/1 -> Pitch actuator fault/3(PitchActFault), Pitch subsystems/2(Fault type 5)

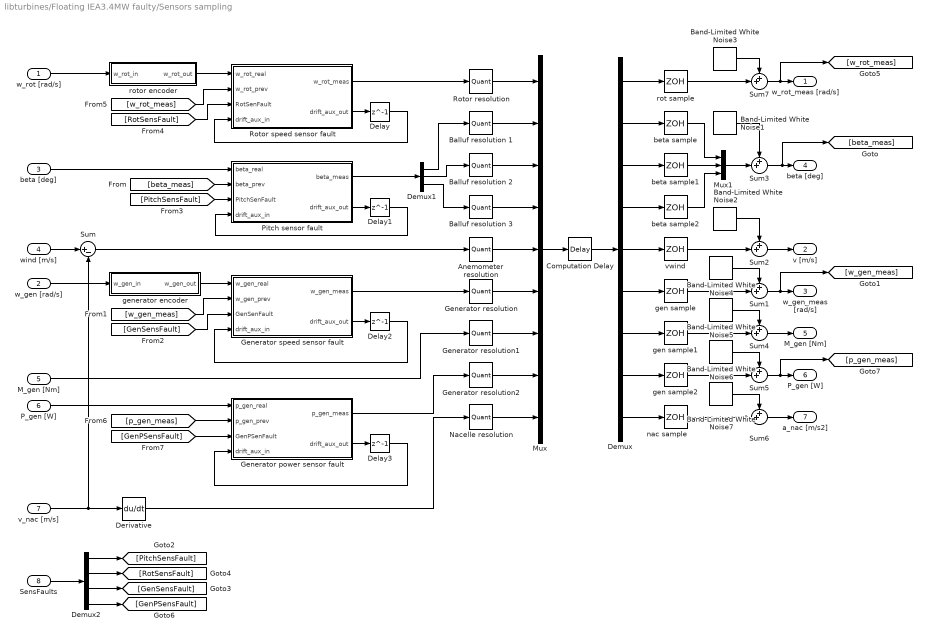
== system libturbines/Floating IEA3.4MW faulty/Sensors sampling ==
  "w_rot [rad/s] " : Inport
  w_gen [rad/s] : Inport  Port=2
  "beta [deg] " : Inport  Port=3
  wind [m/s] : Inport  Port=4
  "M_gen [Nm] " : Inport  Port=5
  "P_gen [W] " : Inport  Port=6
  "v_nac [m/s] " : Inport  Port=7
  SensFaults : Inport  Port=8
  Anemometer resolution : Quantizer  QuantizationInterval=wt.meas.aneres
  Balluf resolution 1 : Quantizer  QuantizationInterval=wt.meas.pitchres
  Balluf resolution 2 : Quantizer  QuantizationInterval=wt.meas.pitchres
  Balluf resolution 3 : Quantizer  QuantizationInterval=wt.meas.pitchres
  Band-Limited White Noise1 : simulink/Sources/Band-Limited White Noise  Cov=noiseFlag*wt.meas.pitchnoise  Ts=dt  seed=floor(10000*rand(1,3))
  Band-Limited White Noise2 : simulink/Sources/Band-Limited White Noise  Cov=noiseFlag*wt.meas.anenoise  Ts=dt  seed=floor(10000*rand(1))
  Band-Limited White Noise3 : simulink/Sources/Band-Limited White Noise  Cov=noiseFlag*wt.meas.rotSpdnoise  Ts=dt  seed=floor(10000*rand(1))
  Band-Limited White Noise4 : simulink/Sources/Band-Limited White Noise  Cov=noiseFlag*wt.meas.genSpdnoise  Ts=dt  seed=floor(10000*rand(1))
  Band-Limited White Noise5 : simulink/Sources/Band-Limited White Noise  Cov=noiseFlag*wt.meas.genTrqnoise  Ts=dt  seed=floor(10000*rand(1))
  Band-Limited White Noise6 : simulink/Sources/Band-Limited White Noise  Cov=noiseFlag*wt.meas.genPwrnoise  Ts=dt  seed=floor(10000*rand(1))
  Band-Limited White Noise7 : simulink/Sources/Band-Limited White Noise  Cov=noiseFlag*wt.meas.nacAccnoise  Ts=dt  seed=floor(10000*rand(1))
  Computation Delay : TransportDelay  DelayTime=wt.meas.delay  InitialOutput=[wt.rotor.ini wt.pitch.ini wt.pitch.ini wt.pitch.ini 0 wt.gen.ini 0 0 0]
  Delay{,1..3} (4 alike) : Delay  DelayLength=1  InitialCondition=0
  Demux : Demux  Outputs=9
  Demux1 : Demux  Outputs=3
  Demux2 : Demux
  Derivative : Derivative
  Generator power sensor fault : MATLAB Function  TreatAsAtomicUnit=on
  Generator resolution : Quantizer  QuantizationInterval=wt.meas.genres
  Generator resolution1 : Quantizer  QuantizationInterval=wt.meas.genres
  Generator resolution2 : Quantizer  QuantizationInterval=wt.meas.genres
  Generator speed sensor fault : MATLAB Function  TreatAsAtomicUnit=on
  Mux : Mux  Inputs=9
  Mux1 : Mux  Inputs=3
  Nacelle resolution : Quantizer  QuantizationInterval=wt.meas.nacres
  Pitch sensor fault : MATLAB Function  TreatAsAtomicUnit=on
  Rotor resolution : Quantizer  QuantizationInterval=wt.meas.rotres
  Rotor speed sensor fault : MATLAB Function  TreatAsAtomicUnit=on
  Sum : Sum  Inputs=|+-
  Sum{1..7} (7 alike) : Sum  Inputs=++|
  beta sample : ZeroOrderHold  SampleTime=wt.meas.Ts
  beta sample1 : ZeroOrderHold  SampleTime=wt.meas.Ts
  beta sample2 : ZeroOrderHold  SampleTime=wt.meas.Ts
  gen sample : ZeroOrderHold  SampleTime=wt.meas.Ts
  gen sample1 : ZeroOrderHold  SampleTime=wt.meas.Ts
  gen sample2 : ZeroOrderHold  SampleTime=wt.meas.Ts
  generator encoder : Subsystem
  nac sample : ZeroOrderHold  SampleTime=wt.meas.Ts
  rot sample : ZeroOrderHold  SampleTime=wt.meas.Ts
  rotor encoder : Subsystem
  vwind : ZeroOrderHold  SampleTime=wt.meas.Ts
  w_rot_meas [rad/s] : Outport  InitialOutput=0
  v [m/s] : Outport  Port=2  InitialOutput=0
  w_gen_meas [rad/s] : Outport  Port=3  InitialOutput=0
  beta [deg] : Outport  Port=4  InitialOutput=0
  M_gen [Nm] : Outport  Port=5  InitialOutput=0
  P_gen [W] : Outport  Port=6  InitialOutput=0
  a_nac [m/s2] : Outport  Port=7  InitialOutput=0
  wires:
  [p_gen_meas] -> Generator power sensor fault/2(p_gen_prev)
  Generator power sensor fault/1(p_gen_meas) -> Generator resolution2/1
  "P_gen [W] "/1 -> Generator power sensor fault/1(p_gen_real)
  Generator power sensor fault/2(drift_aux_out) -> Delay3/1
  [GenPSensFault] -> Generator power sensor fault/3(GenPSenFault)
  Delay3/1 -> Generator power sensor fault/4(drift_aux_in)
  Demux2/4 -> [GenPSensFault]
  wind [m/s]/1 -> Sum/1
  Sum/1 -> Anemometer resolution/1
  Band-Limited White Noise3/1 -> Sum7/1
  Band-Limited White Noise1/1 -> Sum3/1
  Band-Limited White Noise2/1 -> Sum2/1
  Band-Limited White Noise4/1 -> Sum1/1
  Sum7/1 -> w_rot_meas [rad/s]/1, [w_rot_meas]
  rot sample/1 -> Sum7/2
  Sum3/1 -> beta [deg]/1, [beta_meas]
  Mux1/1 -> Sum3/2
  vwind/1 -> Sum2/2
  Sum2/1 -> v [m/s]/1
  gen sample/1 -> Sum1/2
  Sum1/1 -> w_gen_meas [rad/s]/1, [w_gen_meas]
  Demux/9 -> nac sample/1
  Demux/8 -> gen sample2/1
  Demux/7 -> gen sample1/1
  gen sample2/1 -> Sum5/2
  Sum5/1 -> P_gen [W]/1, [p_gen_meas]
  gen sample1/1 -> Sum4/2
  nac sample/1 -> Sum6/2
  Band-Limited White Noise6/1 -> Sum5/1
  Band-Limited White Noise7/1 -> Sum6/1
  Sum6/1 -> a_nac [m/s2]/1
  Sum4/1 -> M_gen [Nm]/1
  Band-Limited White Noise5/1 -> Sum4/1
  Generator resolution2/1 -> Mux/8
  Nacelle resolution/1 -> Mux/9
  Generator resolution1/1 -> Mux/7
  Derivative/1 -> Nacelle resolution/1
  "v_nac [m/s] "/1 -> Sum/2, Derivative/1
  "M_gen [Nm] "/1 -> Generator resolution1/1
  Delay2/1 -> Generator speed sensor fault/4(drift_aux_in)
  Generator speed sensor fault/2(drift_aux_out) -> Delay2/1
  Delay1/1 -> Pitch sensor fault/4(drift_aux_in)
  Pitch sensor fault/2(drift_aux_out) -> Delay1/1
  Delay/1 -> Rotor speed sensor fault/4(drift_aux_in)
  Rotor speed sensor fault/2(drift_aux_out) -> Delay/1
  Demux2/3 -> [GenSensFault]
  Demux2/2 -> [RotSensFault]
  [w_rot_meas] -> Rotor speed sensor fault/2(w_rot_prev)
  [RotSensFault] -> Rotor speed sensor fault/3(RotSenFault)
  [PitchSensFault] -> Pitch sensor fault/3(PitchSenFault)
  [GenSensFault] -> Generator speed sensor fault/3(GenSenFault)
  Demux2/1 -> [PitchSensFault]
  SensFaults/1 -> Demux2/1
  rotor encoder/1(w_rot_out) -> Rotor speed sensor fault/1(w_rot_real)
  Rotor speed sensor fault/1(w_rot_meas) -> Rotor resolution/1
  "w_rot [rad/s] "/1 -> rotor encoder/1(w_rot_in)
  generator encoder/1(w_gen_out) -> Generator speed sensor fault/1(w_gen_real)
  w_gen [rad/s]/1 -> generator encoder/1(w_gen_in)
  [beta_meas] -> Pitch sensor fault/2(beta_prev)
  [w_gen_meas] -> Generator speed sensor fault/2(w_gen_prev)
  Generator speed sensor fault/1(w_gen_meas) -> Generator resolution/1
  Balluf resolution 3/1 -> Mux/4
  Balluf resolution 2/1 -> Mux/3
  Demux/3 -> beta sample1/1
  Demux/4 -> beta sample2/1
  "beta [deg] "/1 -> Pitch sensor fault/1(beta_real)
  Pitch sensor fault/1(beta_meas) -> Demux1/1
  Balluf resolution 1/1 -> Mux/2
  Demux/2 -> beta sample/1
  beta sample2/1 -> Mux1/3
  Demux/1 -> rot sample/1
  beta sample/1 -> Mux1/1
  Demux1/3 -> Balluf resolution 3/1
  Computation Delay/1 -> Demux/1
  Mux/1 -> Computation Delay/1
  Demux/5 -> vwind/1
  Anemometer resolution/1 -> Mux/5
  Demux/6 -> gen sample/1
  Demux1/2 -> Balluf resolution 2/1
  Generator resolution/1 -> Mux/6
  Rotor resolution/1 -> Mux/1
  Demux1/1 -> Balluf resolution 1/1
  beta sample1/1 -> Mux1/2

== system libturbines/Floating IEA3.4MW faulty/Tower deflection  ==
  F_t [N] : Inport
  F_t*h : Gain  Gain=wt.tower.height  SaturateOnIntegerOverflow=on  OutDataTypeStr=Inherit: Same as input  ParamDataTypeStr=Inherit: Same as input
  Tower1 : Subsystem  mask(Tower (thrustwise)){mtop=wt.top.mass, mtow=wt.tower.mass, ftowY=wt.tower.eigfreq, dampY=wt.tower.damp}
      mask prompts: mtop "Mass of towertop [kg]"; mtow "Aequivalent tower mass [kg]"; ftowY "Tower eigenfrequency [Hz]"; dampY "Damping coefficient"
      mask help: Thrustwise dynamics of the tower
      mask init: same as libturbines/Floating IEA15MW/Tower /Tower1
      mask Help: The thrustwise tower dynamics are modelled as a linear oscillator
  v_nac [m/s] : Outport
  M_tow [Nm] : Outport  Port=2
  wires:
  Tower1/1(vnac [m/s]) -> v_nac [m/s]/1
  F_t [N]/1 -> Tower1/1(FT [Nm])
  F_t*h/1 -> M_tow [Nm]/1
  Tower1/2(F_tow [N]) -> F_t*h/1

== system libturbines/Floating NREL5MW/Aerodynamics ==
  note: tip speed
      | [m/s]
  w_rot [rad/s] : Inport
  beta [deg] : Inport  Port=2
  v_rot [m/s] : Inport  Port=3
  C_P & C_T tables1 : $bdroot/Floating NREL5MW faulty/Aerodynamics/Blade 1/C_P & C_T tables  SystemSampleTime=-1  VariantActivationTime=update diagram  EmptyChoice=off  PassThrough=off  PassThroughVariantControl=(default)  EmptyChoiceVariantControl=(default)  AllowFlexibleInterface=on  Latency=0  AutoFrameSizeCalculation=off
  Math Function : Math  Operator=square  SignedPower=on
  Product : Product  InputSameDT=on  SaturateOnIntegerOverflow=on  OutDataTypeStr=Inherit: Same as first input
  Product1 : Product  Inputs=**/  InputSameDT=on  SaturateOnIntegerOverflow=on  OutDataTypeStr=Inherit: Same as first input
  Product2 : Product  InputSameDT=on  SaturateOnIntegerOverflow=on  OutDataTypeStr=Inherit: Same as first input
  Product3 : Product  Inputs=/*  InputSameDT=on  SaturateOnIntegerOverflow=on  OutDataTypeStr=Inherit: Same as first input
  rho/2*A : Gain  Gain=env.rho*.5* pi * wt.rotor.radius^2  SaturateOnIntegerOverflow=on  OutDataTypeStr=Inherit: Same as input  ParamDataTypeStr=Inherit: Same as input
  rotor radius : Gain  Gain=wt.rotor.radius  SaturateOnIntegerOverflow=on  OutDataTypeStr=Inherit: Same as input  ParamDataTypeStr=Inherit: Same as input
  M_rot [Nm] : Outport
  F_t [N] : Outport  Port=2
  C_T : Outport  Port=3
  wires:
  Product2/1 -> Product1/2
  Product1/1 -> M_rot [Nm]/1
  Product/1 -> F_t [N]/1
  beta [deg]/1 -> C_P & C_T tables1/1
  C_P & C_T tables1/2 -> Product1/1
  rotor radius/1 -> Product3/2
  Math Function/1 -> rho/2*A/1
  v_rot [m/s]/1 -> Math Function/1, Product3/1, Product2/1
  w_rot [rad/s]/1 -> rotor radius/1, Product1/3
  Product3/1 -> C_P & C_T tables1/2
  C_P & C_T tables1/1 -> C_T/1, Product/2
  rho/2*A/1 -> Product2/2, Product/1

== system libturbines/Floating NREL5MW/Controller ==
  P_dem [W] : Inport
  w_gen_meas [m/s] : Inport  Port=2
  beta_meas [deg] : Inport  Port=3
  Generator efficiency compensation : Gain  Gain=1/wt.ctrl.gen.effeciency
  Limit power to rated : Saturate  UpperLimit=wt.ctrl.p_rated  LowerLimit=0
  Measurement filter (low pass) : DiscreteStateSpace  A=wt.ctrl.alpha  B=1-wt.ctrl.alpha  C=wt.ctrl.alpha  D=1-wt.ctrl.alpha  InitialCondition=wt.ctrl.gen.ini  SampleTime=wt.ctrl.Ts
  Pitch controller : Subsystem  TreatAsAtomicUnit=on
  Rate Limiter : RateLimiter  RisingSlewLimit=wt.ctrl.torq.ratelim  FallingSlewLimit=-wt.ctrl.torq.ratelim  SampleTimeMode=inherited  InitialCondition=wt.ctrl.torq.ini
  Rated speed : Constant  Value=wt.ctrl.gen.rated
  Region check : Subsystem
  Sample output : ZeroOrderHold  SampleTime=wt.ctrl.Ts
  Sample power demand : ZeroOrderHold  SampleTime=wt.ctrl.Ts
  Saturation : Saturate  UpperLimit=wt.ctrl.torq.lim  LowerLimit=0
  Sum : Sum  Inputs=+-|
  Torque - speed lookup table : Lookup  InputValues=wt.ctrl.torq.wg  Table=wt.ctrl.torq.M  LookUpMeth=Interpolation-Use End Values  SaturateOnIntegerOverflow=off
  Zero-Order Hold : ZeroOrderHold  SampleTime=wt.ctrl.Ts
  beta_ref [deg] : Outport
  M_g_ref [W] : Outport  Port=2
  wires:
  beta_meas [deg]/1 -> Pitch controller/3(beta_meas [deg])
  Pitch controller/1(beta_ref [deg]) -> Region check/4(pitch command), Zero-Order Hold/1
  w_gen_meas [m/s]/1 -> Measurement filter (low pass)/1
  Measurement filter (low pass)/1 -> Torque - speed lookup table/1, Region check/2(w_gen), Sum/2  "Filtered generator speed"
  Saturation/1 -> Rate Limiter/1
  Torque - speed lookup table/1 -> Region check/1(Torque_dem)  "Desired Torque"
  P_dem [W]/1 -> Sample power demand/1
  Region check/1(Torque_ref) -> Saturation/1
  Limit power to rated/1 -> Pitch controller/2(P_dem), Region check/3(p_dem)
  Zero-Order Hold/1 -> beta_ref [deg]/1
  Sample output/1 -> M_g_ref [W]/1
  Generator efficiency compensation/1 -> Limit power to rated/1
  Rate Limiter/1 -> Sample output/1
  Sample power demand/1 -> Generator efficiency compensation/1
  Rated speed/1 -> Sum/1
  Sum/1 -> Pitch controller/1(w_gen_diff)
  Region check/2(Enable pitch controller) -> Pitch controller/Enable

== system libturbines/Floating NREL5MW/Drive Train ==
  M_rot [Nm] : Inport
  M_gen [Nm] : Inport  Port=2
  Demux : Demux  Outputs=3
  Drive train dynamics : StateSpace  A=wt.dt.ssA  B=wt.dt.ssB  C=wt.dt.ssC  D=wt.dt.ssD  InitialCondition=[wt.rotor.ini;wt.gen.ini;0]
  Mux : Mux  Inputs=2
  w_rot [rad/s] : Outport
  w_gen [rad/s] : Outport  Port=2
  M_shaft [Nm] : Outport  Port=3
  wires:
  Demux/3 -> M_shaft [Nm]/1
  Demux/2 -> w_gen [rad/s]/1
  Demux/1 -> w_rot [rad/s]/1
  Drive train dynamics/1 -> Demux/1
  M_gen [Nm]/1 -> Mux/2
  M_rot [Nm]/1 -> Mux/1
  Mux/1 -> Drive train dynamics/1

== system libturbines/Floating NREL5MW/Generator simple ==
  w_gen [rad/s] : Inport
  M_g_ref [W] : Inport  Port=2
  Constant : Constant  Value=wt.gen.timeconstant
  Divide1 : Product  Inputs=*/
  Generator efficiency : Gain  Gain=wt.gen.effeciency
  Multiply : Product  Inputs=**
  Sum : Sum  Inputs=|+-
  Torque Integrator : Integrator  InitialCondition=wt.gen.torq.ini
  M_gen [Nm] : Outport
  P_out [W] : Outport  Port=2
  wires:
  Sum/1 -> Divide1/1
  Torque Integrator/1 -> Multiply/1, Sum/2, M_gen [Nm]/1
  w_gen [rad/s]/1 -> Multiply/2
  M_g_ref [W]/1 -> Sum/1
  Multiply/1 -> Generator efficiency/1
  Generator efficiency/1 -> P_out [W]/1
  Divide1/1 -> Torque Integrator/1
  Constant/1 -> Divide1/2

== system libturbines/Floating NREL5MW/Hydrodynamics ==
  F_t [N] : Inport
  F_ex : Inport  Port=2
  Gain : Gain  Gain=plat.nF2pT  Multiplication=Matrix(K*u)
  Gain2 : Gain  Gain=plat.pM2nM_surge  Multiplication=Matrix(K*u)
  Gain3 : Gain  Gain=plat.pM2nM_pitch  Multiplication=Matrix(K*u)
  Platform hydrodynamics SS system : StateSpace  A=plat.HydSys.a  B=plat.HydSys.b  C=plat.HydSys.c  D=plat.HydSys.d  InitialCondition=0
  Sum : Sum  Inputs=++|
  Sum2 : Sum  Inputs=+|+
  v_nac_hyd [m/s] : Outport
  wires:
  F_t [N]/1 -> Gain/1
  Gain/1 -> Sum/1
  Gain3/1 -> Sum2/2
  Gain2/1 -> Sum2/1
  Platform hydrodynamics SS system/1 -> Gain2/1, Gain3/1
  Sum2/1 -> v_nac_hyd [m/s]/1
  Sum/1 -> Platform hydrodynamics SS system/1
  F_ex/1 -> Sum/2

== system libturbines/Floating NREL5MW/Pitch Actuator ==
  beta_ref [deg] : Inport
  Pitch system : StateSpace  A=wt.pitch.ssA  B=wt.pitch.ssB  C=wt.pitch.ssC  D=wt.pitch.ssD  InitialCondition=0
  beta [deg] : Outport
  wires:
  Pitch system/1 -> beta [deg]/1
  beta_ref [deg]/1 -> Pitch system/1

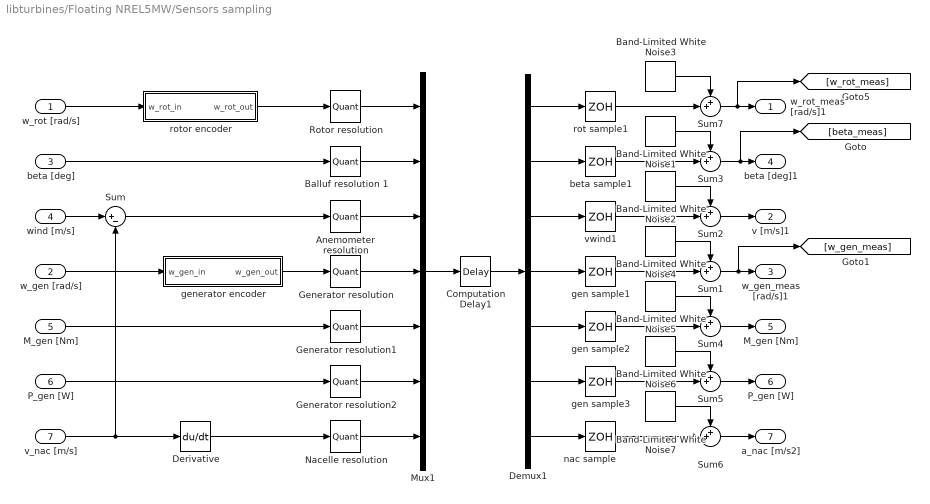
== system libturbines/Floating NREL5MW/Sensors sampling ==
  "w_rot [rad/s] " : Inport
  w_gen [rad/s] : Inport  Port=2
  "beta [deg] " : Inport  Port=3
  wind [m/s] : Inport  Port=4
  "M_gen [Nm] " : Inport  Port=5
  "P_gen [W] " : Inport  Port=6
  "v_nac [m/s] " : Inport  Port=7
  Anemometer resolution : Quantizer  QuantizationInterval=wt.meas.aneres
  Balluf resolution 1 : Quantizer  QuantizationInterval=wt.meas.pitchres
  Band-Limited White Noise1 : simulink/Sources/Band-Limited White Noise  Cov=noiseFlag*wt.meas.pitchnoise  Ts=dt  seed=floor(10000*rand(1))
  Band-Limited White Noise2 : simulink/Sources/Band-Limited White Noise  Cov=noiseFlag*wt.meas.anenoise  Ts=dt  seed=floor(10000*rand(1))
  Band-Limited White Noise3 : simulink/Sources/Band-Limited White Noise  Cov=noiseFlag*wt.meas.rotSpdnoise  Ts=dt  seed=floor(10000*rand(1))
  Band-Limited White Noise4 : simulink/Sources/Band-Limited White Noise  Cov=noiseFlag*wt.meas.genSpdnoise  Ts=dt  seed=floor(10000*rand(1))
  Band-Limited White Noise5 : simulink/Sources/Band-Limited White Noise  Cov=noiseFlag*wt.meas.genTrqnoise  Ts=dt  seed=floor(10000*rand(1))
  Band-Limited White Noise6 : simulink/Sources/Band-Limited White Noise  Cov=noiseFlag*wt.meas.genPwrnoise  Ts=dt  seed=floor(10000*rand(1))
  Band-Limited White Noise7 : simulink/Sources/Band-Limited White Noise  Cov=noiseFlag*wt.meas.nacAccnoise  Ts=dt  seed=floor(10000*rand(1))
  Computation Delay1 : TransportDelay  DelayTime=wt.meas.delay  InitialOutput=[wt.rotor.ini wt.pitch.ini 0 wt.gen.ini 0 0 0]
  Demux1 : Demux  Outputs=7
  Derivative : Derivative
  Generator resolution : Quantizer  QuantizationInterval=wt.meas.genres
  Generator resolution1 : Quantizer  QuantizationInterval=wt.meas.genres
  Generator resolution2 : Quantizer  QuantizationInterval=wt.meas.genres
  Mux1 : Mux  Inputs=7
  Nacelle resolution : Quantizer  QuantizationInterval=wt.meas.nacres
  Rotor resolution : Quantizer  QuantizationInterval=wt.meas.rotres
  Sum : Sum  Inputs=|+-
  Sum{1..7} (7 alike) : Sum  Inputs=++|
  beta sample1 : ZeroOrderHold  SampleTime=wt.meas.Ts
  gen sample1 : ZeroOrderHold  SampleTime=wt.meas.Ts
  gen sample2 : ZeroOrderHold  SampleTime=wt.meas.Ts
  gen sample3 : ZeroOrderHold  SampleTime=wt.meas.Ts
  generator encoder : Subsystem
  nac sample : ZeroOrderHold  SampleTime=wt.meas.Ts
  rot sample1 : ZeroOrderHold  SampleTime=wt.meas.Ts
  rotor encoder : Subsystem
  vwind1 : ZeroOrderHold  SampleTime=wt.meas.Ts
  w_rot_meas [rad/s]1 : Outport  InitialOutput=0
  v [m/s]1 : Outport  Port=2  InitialOutput=0
  w_gen_meas [rad/s]1 : Outport  Port=3  InitialOutput=0
  beta [deg]1 : Outport  Port=4  InitialOutput=0
  M_gen [Nm] : Outport  Port=5  InitialOutput=0
  P_gen [W] : Outport  Port=6  InitialOutput=0
  a_nac [m/s2] : Outport  Port=7  InitialOutput=0
  wires:
  rotor encoder/1(w_rot_out) -> Rotor resolution/1
  "w_rot [rad/s] "/1 -> rotor encoder/1(w_rot_in)
  w_gen [rad/s]/1 -> generator encoder/1(w_gen_in)
  generator encoder/1(w_gen_out) -> Generator resolution/1
  Rotor resolution/1 -> Mux1/1
  "beta [deg] "/1 -> Balluf resolution 1/1
  Computation Delay1/1 -> Demux1/1
  beta sample1/1 -> Sum3/2
  Demux1/1 -> rot sample1/1
  Demux1/2 -> beta sample1/1
  Band-Limited White Noise7/1 -> Sum6/1
  Band-Limited White Noise6/1 -> Sum5/1
  Sum2/1 -> v [m/s]1/1
  Sum3/1 -> [beta_meas], beta [deg]1/1
  Mux1/1 -> Computation Delay1/1
  rot sample1/1 -> Sum7/2
  Band-Limited White Noise3/1 -> Sum7/1
  gen sample1/1 -> Sum1/2
  Band-Limited White Noise5/1 -> Sum4/1
  Band-Limited White Noise4/1 -> Sum1/1
  Sum7/1 -> [w_rot_meas], w_rot_meas [rad/s]1/1
  vwind1/1 -> Sum2/2
  Sum6/1 -> a_nac [m/s2]/1
  Sum4/1 -> M_gen [Nm]/1
  nac sample/1 -> Sum6/2
  Band-Limited White Noise1/1 -> Sum3/1
  gen sample3/1 -> Sum5/2
  Sum5/1 -> P_gen [W]/1
  Sum1/1 -> [w_gen_meas], w_gen_meas [rad/s]1/1
  gen sample2/1 -> Sum4/2
  Band-Limited White Noise2/1 -> Sum2/1
  Balluf resolution 1/1 -> Mux1/2
  Anemometer resolution/1 -> Mux1/3
  Generator resolution/1 -> Mux1/4
  "v_nac [m/s] "/1 -> Sum/2, Derivative/1
  Demux1/7 -> nac sample/1
  Demux1/6 -> gen sample3/1
  Demux1/5 -> gen sample2/1
  Demux1/4 -> gen sample1/1
  Demux1/3 -> vwind1/1
  Generator resolution1/1 -> Mux1/5
  Generator resolution2/1 -> Mux1/6
  Nacelle resolution/1 -> Mux1/7
  Derivative/1 -> Nacelle resolution/1
  "P_gen [W] "/1 -> Generator resolution2/1
  "M_gen [Nm] "/1 -> Generator resolution1/1
  wind [m/s]/1 -> Sum/1
  Sum/1 -> Anemometer resolution/1

== system libturbines/Floating NREL5MW/Tower  ==
  F_t [N] : Inport
  F_t*h : Gain  Gain=wt.tower.height  SaturateOnIntegerOverflow=on  OutDataTypeStr=Inherit: Same as input  ParamDataTypeStr=Inherit: Same as input
  Tower1 : Subsystem  mask(Tower (thrustwise)){mtop=wt.top.mass, mtow=wt.tower.mass, ftowY=wt.tower.eigfreq, dampY=wt.tower.damp}
      mask prompts: mtop "Mass of towertop [kg]"; mtow "Aequivalent tower mass [kg]"; ftowY "Tower eigenfrequency [Hz]"; dampY "Damping coefficient"
      mask help: Thrustwise dynamics of the tower
      mask init: same as libturbines/Floating IEA15MW/Tower /Tower1
      mask Help: The thrustwise tower dynamics are modelled as a linear oscillator
  M_tow [Nm] : Outport
  v_nac [m/s] : Outport  Port=2
  wires:
  Tower1/1(vnac [m/s]) -> v_nac [m/s]/1
  F_t [N]/1 -> Tower1/1(FT [Nm])
  F_t*h/1 -> M_tow [Nm]/1
  Tower1/2(F_tow [N]) -> F_t*h/1

== system libturbines/Floating NREL5MW faulty/Aerodynamics ==
  w_rot [rad/s] : Inport
  beta [deg] : Inport  Port=2
  v_rot [m/s] : Inport  Port=3
  Blade 1 : Subsystem
  Blade 2 : Subsystem  AncestorBlock=libturbines/Floating faulty NREL5MW1/Aerodynamics/Blade 1
  Blade 3 : Subsystem  AncestorBlock=libturbines/Floating faulty NREL5MW1/Aerodynamics/Blade 1
  Demux : Demux  Outputs=3
  Sum : Sum  Inputs=+++
  Sum1 : Sum  Inputs=+++
  Sum2 : Sum  Inputs=+++
  M_rot [Nm] : Outport
  F_t [N] : Outport  Port=2
  C_T : Outport  Port=3
  wires:
  v_rot [m/s]/1 -> Blade 3/1(v_rot [m/s]), Blade 2/1(v_rot [m/s]), Blade 1/1(v_rot [m/s])
  w_rot [rad/s]/1 -> Blade 3/3(w_rot [rad/s]), Blade 2/3(w_rot [rad/s]), Blade 1/3(w_rot [rad/s])
  Sum/1 -> F_t [N]/1
  Sum2/1 -> M_rot [Nm]/1
  Sum1/1 -> C_T/1
  Blade 2/3(M_rot [Nm]) -> Sum2/2
  Blade 3/3(M_rot [Nm]) -> Sum2/3
  Blade 3/1(F_t [N]) -> Sum/3
  Blade 3/2(C_T) -> Sum1/3
  Blade 1/3(M_rot [Nm]) -> Sum2/1
  Blade 1/1(F_t [N]) -> Sum/1
  Blade 1/2(C_T) -> Sum1/1
  Blade 2/1(F_t [N]) -> Sum/2
  Blade 2/2(C_T) -> Sum1/2
  beta [deg]/1 -> Demux/1
  Demux/1 -> Blade 1/2(beta [deg])
  Demux/3 -> Blade 3/2(beta [deg])
  Demux/2 -> Blade 2/2(beta [deg])
